simulink library "BrickPiSimSubLib_Read"  (R2019a)
settings: Solver=VariableStepAuto  StartTime=0.0  StopTime=10.0  RelTol=1e-3
undefined symbols (not defined in the file or in its folder): Ts
libraries: hdlsllib x4, $bdroot x2, raspberrypilib x2, simulink x1
settings Model: Creator=hahn  LastModifiedBy=uk008555

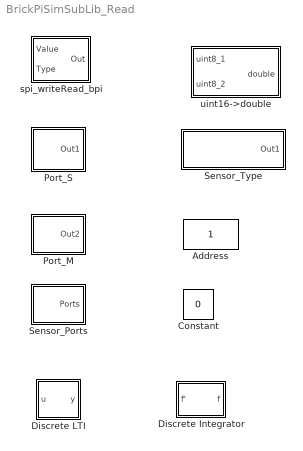
== system BrickPiSimSubLib_Read ==
  Address : Constant  OutDataTypeStr=uint8  mask{Add_Val=1}
      mask prompts: Add_Val "SPI Address"
      mask init:
      | add_val=Add_Val;
      mask Display: disp(['Address: ' num2str(add_val)])
  Constant : Constant  Value=0  OutDataTypeStr=uint8
  Discrete Integrator : Subsystem
      mask Display: disp('s^-1')
  Discrete LTI : Subsystem  mask{A=1, B=1, C=1, D=1}
  Port_M : Subsystem  mask{Port_Val=A}
      mask prompts: Port_Val "Port"
      mask init:
      | port_val=Port_Val;
      | switch Port_Val
      |     case 1
      |         port_val='A';
      |     case 2
      |         port_val='B';
      |     case 3
      |         port_val='C';
      |     case 4
      |         port_val='D';
      |     otherwise
      |         port_val='failure';
      | end
      mask TypeOptions Port_Val: A | B | C | D
      mask Display: disp(['Motor: ',num2str(port_val)])
  Port_S : Subsystem  mask{Port_Val=1}
      mask prompts: Port_Val "Port"
      mask init:
      | port_val=Port_Val;
      mask TypeOptions Port_Val: 1 | 2 | 3 | 4
      mask Display: disp(['Sensor: ',num2str(port_val)])
  Sensor_Ports : Subsystem  mask{Port1_Val=off, Port2_Val=on, Port3_Val=off, Port4_Val=on}
      mask prompts: Port1_Val "Port1"; Port2_Val "Port2"; Port3_Val "Port3"; Port4_Val "Port4"
  Sensor_Type : Subsystem  mask{Type_Val=None}
      mask prompts: Type_Val "Sensor Type:"
      mask init:
      | switch Type_Val
      |     case 1
      |         type_val='None';
      |     case 15
      |         type_val='Gyro ABS';
      |     case 16
      |         type_val='Gyro DPS';
      |     case 17
      |         type_val='Gyro ABS & DPS';
      |     otherwise
      |         type_val=['Sensor Type: ' num2str(Type_Val)];
      | end
      mask TypeOptions Type_Val: None | I2C | Custom | Touch | Touch NXT | Touch EV3 | NXT Light on | NXT Light off | NXT Color Red | NXT Color Green | NXT Color Blue | NXT Color Full | NXT Color Off | NXT Ultrasonic | Ev3 Gyro ABS | Ev3 Gyro DPS | Ev3 ABS & DPS
      mask Display: disp(type_val)
  spi_writeRead_bpi : Subsystem  mask{Add_Val=1, Port_Val=1}
      mask prompts: Add_Val "SPI Address"; Port_Val "Port"
      mask TypeOptions Add_Val: Address/Add_Val
      mask TypeOptions Port_Val: Port_S/Port_Val
  uint16->double : Subsystem

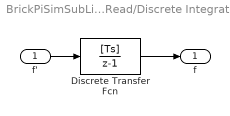
== system BrickPiSimSubLib_Read/Discrete Integrator ==
  f' : Inport
  Discrete Transfer Fcn : DiscreteTransferFcn  Numerator=[Ts]  Denominator=[1 -1]
  f : Outport
  wires:
  f'/1 -> Discrete Transfer Fcn/1
  Discrete Transfer Fcn/1 -> f/1

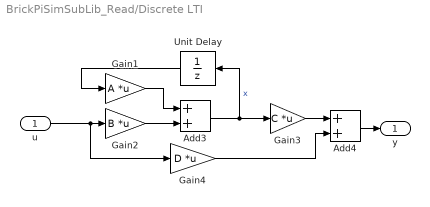
== system BrickPiSimSubLib_Read/Discrete LTI ==
  u : Inport
  Add3 : Sum
  Add4 : Sum
  Gain1 : Gain  Gain=A  Multiplication=Matrix(K*u)
  Gain2 : Gain  Gain=B  Multiplication=Matrix(K*u)
  Gain3 : Gain  Gain=C  Multiplication=Matrix(K*u)
  Gain4 : Gain  Gain=D  Multiplication=Matrix(K*u)
  Unit Delay : UnitDelay  SampleTime=-1  HasFrameUpgradeWarning=on
  y : Outport
  wires:
  Gain4/1 -> Add4/2
  Gain1/1 -> Add3/1
  Add4/1 -> y/1
  u/1 -> Gain2/1, Gain4/1
  Add3/1 -> Unit Delay/1, Gain3/1  "x"
  Gain2/1 -> Add3/2
  Gain3/1 -> Add4/1
  Unit Delay/1 -> Gain1/1

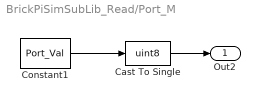
== system BrickPiSimSubLib_Read/Port_M ==
  Cast To Single : DataTypeConversion  OutDataTypeStr=uint8
  Constant1 : Constant  Value=Port_Val
  Out2 : Outport
  wires:
  Cast To Single/1 -> Out2/1
  Constant1/1 -> Cast To Single/1

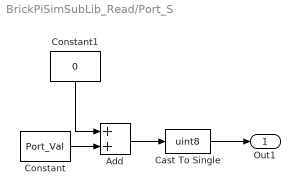
== system BrickPiSimSubLib_Read/Port_S ==
  Add : Sum
  Cast To Single : DataTypeConversion  OutDataTypeStr=uint8
  Constant : Constant  Value=Port_Val
  Constant1 : Constant  Value=0
  Out1 : Outport
  wires:
  Constant1/1 -> Add/1
  Add/1 -> Cast To Single/1
  Constant/1 -> Add/2
  Cast To Single/1 -> Out1/1

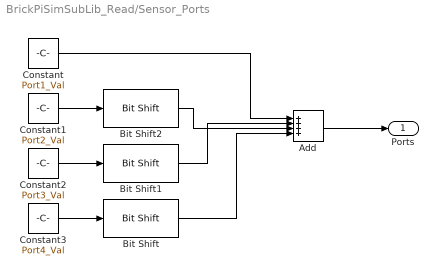
== system BrickPiSimSubLib_Read/Sensor_Ports ==
  Add : Sum  Inputs=++++
  Bit Shift : hdlsllib/Logic and Bit Operations/Bit Shift  mode=Shift Left Logical  N=3
      settings: SourceProductName=Simulink
  Bit Shift1 : hdlsllib/Logic and Bit Operations/Bit Shift  mode=Shift Left Logical  N=2
      settings: SourceProductName=Simulink
  Bit Shift2 : hdlsllib/Logic and Bit Operations/Bit Shift  mode=Shift Left Logical  N=1
      settings: SourceProductName=Simulink
  Constant : Constant  Value=Port1_Val  OutDataTypeStr=uint8
  Constant1 : Constant  Value=Port2_Val  OutDataTypeStr=uint8
  Constant2 : Constant  Value=Port3_Val  OutDataTypeStr=uint8
  Constant3 : Constant  Value=Port4_Val  OutDataTypeStr=uint8
  Ports : Outport
  wires:
  Constant3/1 -> Bit Shift/1
  Constant2/1 -> Bit Shift1/1
  Constant/1 -> Add/1
  Bit Shift/1 -> Add/4
  Constant1/1 -> Bit Shift2/1
  Add/1 -> Ports/1
  Bit Shift2/1 -> Add/3
  Bit Shift1/1 -> Add/2

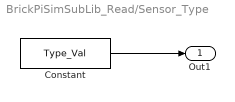
== system BrickPiSimSubLib_Read/Sensor_Type ==
  Constant : Constant  Value=Type_Val  OutDataTypeStr=uint8
  Out1 : Outport
  wires:
  Constant/1 -> Out1/1

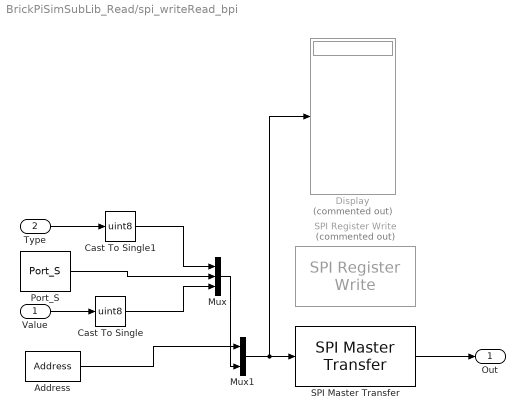
== system BrickPiSimSubLib_Read/spi_writeRead_bpi ==
  Value : Inport
  Type : Inport  Port=2
  Address : $bdroot/Address  Add_Val=Add_Val
  Cast To Single : DataTypeConversion  OutDataTypeStr=uint8
  Cast To Single1 : DataTypeConversion  OutDataTypeStr=uint8
  Display : Display  Commented=on
  Mux : Mux  Inputs=3
  Mux1 : Mux  Inputs=2
  Port_S : $bdroot/Port_S  Port_Val=1
  SPI Master Transfer : raspberrypilib/SPI Master Transfer  BoardProperty=Pi 3 Model B+  SPIModule=uint32(0)  Mode=Master  BusSpeed=1000000  Pin=SPI0_CE1  FirstBitToTransfer=Most significant bit (MSB)  ClockMode=0  BlockFunction=Transfer  RegisterAddress=0  OutputDataType=int8  OutputDataLength=1
      settings: SourceProductName=Simulink Support Package for Raspberry Pi Hardware  SourceProductBaseCode=RASPPI
  SPI Register Write : raspberrypilib/SPI Register Write  Commented=on  BoardProperty=Pi 3 Model B+  SPIModule=uint32(0)  Mode=Master  BusSpeed=1000000  Pin=SPI0_CE1  FirstBitToTransfer=Most significant bit (MSB)  ClockMode=0  BlockFunction=Write  RegisterAddress=0  OutputDataType=int8  OutputDataLength=1
      settings: SourceProductName=Simulink Support Package for Raspberry Pi Hardware  SourceProductBaseCode=RASPPI
  Out : Outport
  wires:
  Value/1 -> Cast To Single/1
  Cast To Single/1 -> Mux/3
  Mux/1 -> Mux1/2
  Port_S/1 -> Mux/2
  Type/1 -> Cast To Single1/1
  Address/1 -> Mux1/1
  SPI Master Transfer/1 -> Out/1
  Mux1/1 -> Display/1, SPI Master Transfer/1
  Cast To Single1/1 -> Mux/1

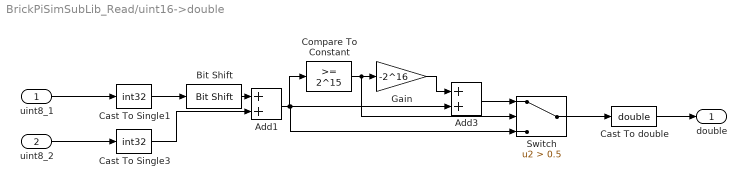
== system BrickPiSimSubLib_Read/uint16->double ==
  uint8_1 : Inport
  uint8_2 : Inport  Port=2
  Add1 : Sum
  Add3 : Sum
  Bit Shift : hdlsllib/Logic and Bit Operations/Bit Shift  mode=Shift Left Logical  N=8
      settings: SourceProductName=Simulink
  Cast To Single1 : DataTypeConversion  OutDataTypeStr=int32
  Cast To Single3 : DataTypeConversion  OutDataTypeStr=int32
  Cast To double : DataTypeConversion  OutDataTypeStr=double
  Compare To Constant : simulink/Logic and Bit Operations/Compare To Constant  relop=>=  const=2^15  OutDataTypeStr=boolean
  Gain : Gain  Gain=-2^16
  Switch : Switch  Criteria=u2 > Threshold  Threshold=0.5
  double : Outport
  wires:
  Cast To Single1/1 -> Bit Shift/1
  uint8_2/1 -> Cast To Single3/1
  Add1/1 -> Switch/3, Add3/2, Compare To Constant/1
  Bit Shift/1 -> Add1/1
  Gain/1 -> Add3/1
  uint8_1/1 -> Cast To Single1/1
  Switch/1 -> Cast To double/1
  Cast To Single3/1 -> Add1/2
  Cast To double/1 -> double/1
  Compare To Constant/1 -> Switch/2, Gain/1
  Add3/1 -> Switch/1
